simulink model "pha_0_9_signal"  (R2023a)
settings: Solver=VariableStepAuto  StartTime=0.0  StopTime=1000  RelTol=1e-3
settings Model: Creator=Dovlica  LastModifiedBy=Dovlica
settings SimscapeCC: SimscapeLogType=all

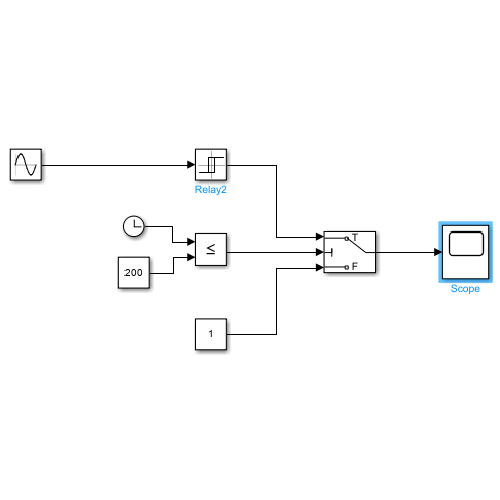
[thumbnail: Simulink's stored preview of the top-level diagram]
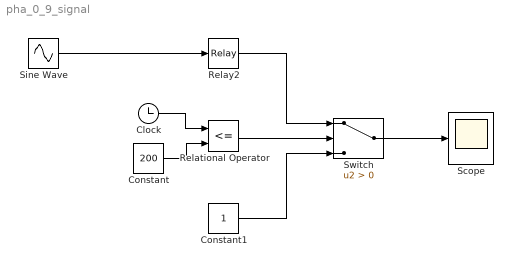
== system pha_0_9_signal ==
  Clock : Clock
  Constant : Constant  Value=200
  Constant1 : Constant
  Relational Operator : RelationalOperator  Operator=<=  OutDataTypeStr=boolean  RndMeth=Simplest  InputSameDT=off
  Relay2 : Relay  OnSwitchValue=5  OffSwitchValue=4.5  OnOutputValue=-1  OffOutputValue=1
  Scope : Scope
  Sine Wave : Sin  Amplitude=0.75  Bias=4.75  SampleTime=0
  Switch : Switch  Criteria=u2 > Threshold  SaturateOnIntegerOverflow=off  InputSameDT=off
  wires:
  Relay2/1 -> Switch/1
  Sine Wave/1 -> Relay2/1
  Clock/1 -> Relational Operator/1
  Constant/1 -> Relational Operator/2
  Relational Operator/1 -> Switch/2
  Constant1/1 -> Switch/3
  Switch/1 -> Scope/1
